simulink model "simulation1"  (R2014b)
settings: Solver=ode45  StartTime=0.0  StopTime=10  RelTol=1e-3
values from neighbouring files (symbols this model uses):
  k = 100    [deloppgave_j.m]    (also in main1.m; main2.m = 6; main_i.m)
  m = 200    [deloppgave_j.m]    (also in main1.m; main2.m = 2; main_i.m)
  v_0 = v(end)    [deloppgave_j.m]    (also in main1.m = 0; main_i.m = xVec1(end))
settings Model: Creator=rende_000  LastModifiedBy=rende_000

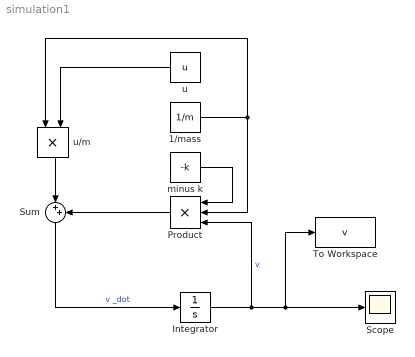
== system simulation1 ==
  1/mass : Constant  Value=1/m
  Integrator : Integrator  InitialCondition=v_0
  Product : Product  Inputs=3
  Scope : Scope
  Sum : Sum  Inputs=|++
  To Workspace : ToWorkspace  VariableName=v  SaveFormat=Timeseries  SampleTime=-1
  minus k : Constant  Value=-k
  u : Constant  Value=u
  u/m : Product
  wires:
  Sum/1 -> Integrator/1  "v _dot"
  Integrator/1 -> To Workspace/1, Scope/1, Product/3  "v"
  1/mass/1 -> Product/2, u/m/1
  minus k/1 -> Product/1
  u/1 -> u/m/2
  u/m/1 -> Sum/1
  Product/1 -> Sum/2
